simulink model "Room_Thermal_Baseline"  (R2021a)
settings: Solver=VariableStepAuto  StartTime=0.0  StopTime=2592000  RelTol=1e-3
libraries: simulink x1
settings Model: Creator=OGHOSA  LastModifiedBy=OGHOSA

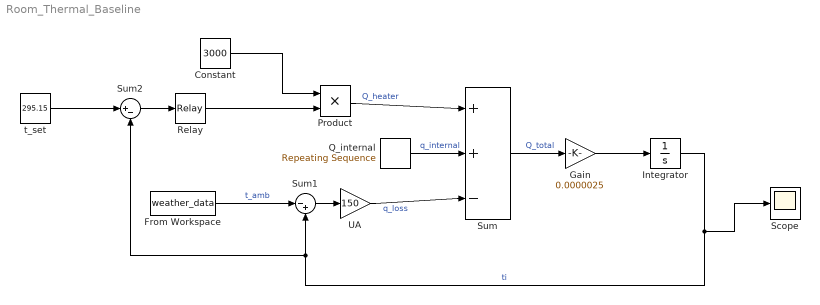
== system Room_Thermal_Baseline ==
  Constant : Constant  Value=3000
  From Workspace : FromWorkspace  VariableName=weather_data
  Gain : Gain  Gain=0.0000025
  Integrator : Integrator  InitialCondition=293.15
  Product : Product
  Q_internal : simulink/Sources/Repeating Sequence  rep_seq_t=[0, 28000, 64000, 86400]  rep_seq_y=[100, 500, 100, 100]
  Relay : Relay  OnSwitchValue=1  OffSwitchValue=-1
  Scope : Scope
  Sum : Sum  Inputs=+|+|-
  Sum1 : Sum  Inputs=|-+
  Sum2 : Sum  Inputs=|+-
  UA : Gain  Gain=150
  t_set : Constant  Value=295.15
  wires:
  Sum/1 -> Gain/1  "Q_total"
  Gain/1 -> Integrator/1
  Q_internal/1 -> Sum/2  "q_internal"
  Integrator/1 -> Scope/1, Sum2/2, Sum1/2  "ti"
  Sum1/1 -> UA/1
  UA/1 -> Sum/3  "q_loss"
  Product/1 -> Sum/1  "Q_heater"
  From Workspace/1 -> Sum1/1  "t_amb"
  t_set/1 -> Sum2/1
  Sum2/1 -> Relay/1
  Relay/1 -> Product/2
  Constant/1 -> Product/1
